simulink model "fbd1"  (R2022b)
settings: Solver=VariableStepAuto  StartTime=0.0  StopTime=150  RelTol=1e-3
settings Model: Creator=Asus  LastModifiedBy=Asus

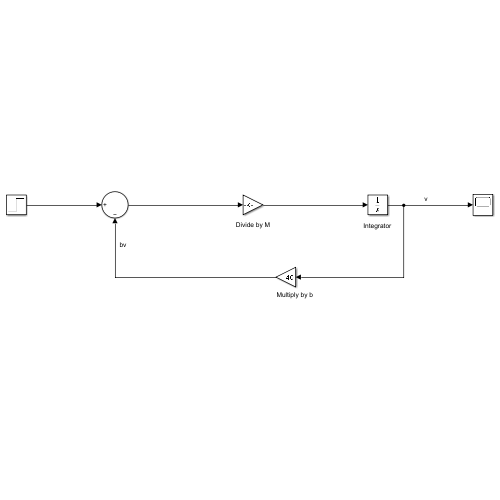
[thumbnail: Simulink's stored preview of the top-level diagram]
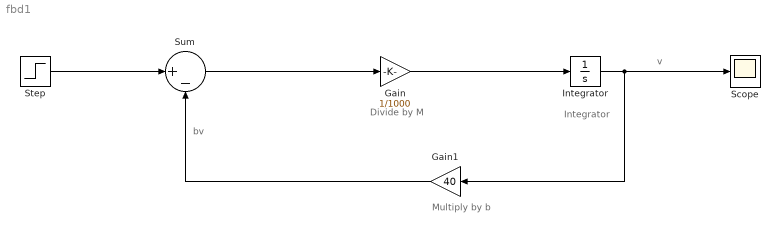
== system fbd1 ==
  note: Multiply by b
  note: v
  note: Integrator
  note: Divide by M
  note: bv
  Gain : Gain  Gain=1/1000
  Gain1 : Gain  Gain=40
  Integrator : Integrator
  Scope : Scope
  Step : Step  After=400  SampleTime=0
  Sum : Sum  Inputs=|+-
  wires:
  Sum/1 -> Gain/1
  Gain/1 -> Integrator/1
  Integrator/1 -> Scope/1, Gain1/1
  Gain1/1 -> Sum/2
  Step/1 -> Sum/1
